simulink model "sysgenIIR_DFormI_dp"  (Simulink 7.6)
settings: Solver=VariableStepDiscrete  SolverMode=SingleTasking  StartTime=0.0  StopTime=20000  RelTol=1e-3
PreLoadFcn:
  | xlrequire('PreLoadFcn')
values from neighbouring files (symbols this model uses):
  Fs = 1 ./ block_data.params.XIncr    [sdspfscope2_r13.m]
undefined symbols (not defined in the file or in its folder): a1, a2, b0, b1, b2, One, sided
libraries: xbsIndex_r4 x46, dspobslib x3, dspsnks4 x3, dspstat3 x2, simulink x2, xbsCopyrightNotice_r4 x1, dspswit3 x1, dspsrcs4 x1
settings Model: Creator=alexc  LastModifiedBy=douangp
settings DataIOCC: SignalLoggingName=sigsOut
settings OptimizationCC: BlockReduction=off  BooleanDataType=off  InlineInvariantSignals=on  InitFltsAndDblsToZero=on
settings DebuggingCC: SaveWithParameterizedLinksMsg=none  SignalResolutionControl=TryResolveAllWithWarning  SolverPrmCheckMsg=none  MultiTaskDSMMsg=warning  MultiTaskCondExecSysMsg=none  StrictBusMsg=None
settings HardwareCC: TargetUnknown=on
settings RTWCC: IncludeERTFirstTime=on
settings GRTTargetCC: TargetFcnLib=ansi_tfl_tmw.mat

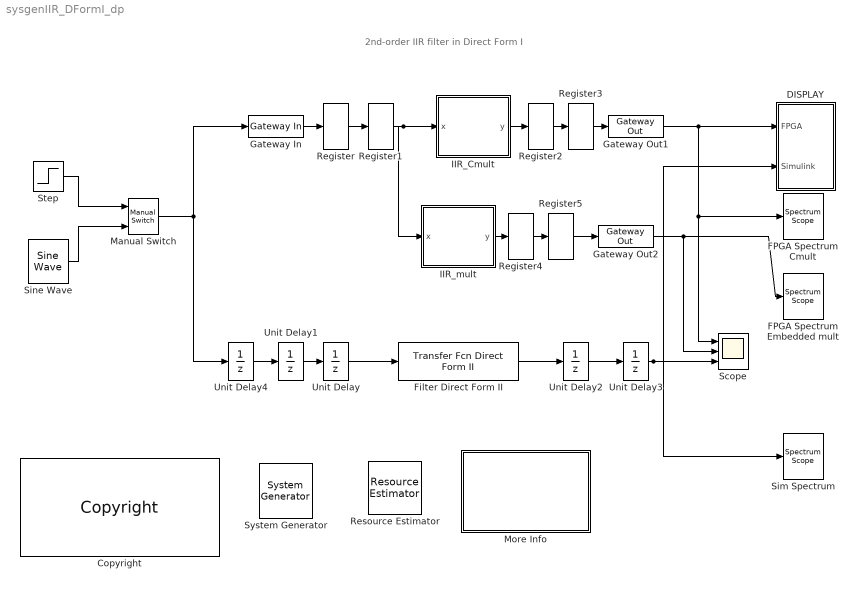
== system sysgenIIR_DFormI_dp ==
  note: 2nd-order IIR filter in Direct Form I
  " System Generator" : xbsIndex_r4/ System Generator  Tag=genX  SystemSampleTime=-1  xilinxfamily=virtex6  part=xc6vlx240t  speed=-1  package=ff1156  synthesis_tool=XST  clock_wrapper=Clock Enables  directory=./sysgenIIR_DFormI_work_registered  testbench=on  simulink_period=Fs  sysclk_period=16  dcm_input_clock_period=100  incr_netlist=off  trim_vbits=According to Block Masks  dbl_ovrd=According to Block Masks  core_generation=According to Block Masks  run_coregen=off  deprecated_control=off  eval_field=0  block_type=sysgen
      settings: block_version=9.2.00
  Copyright : xbsCopyrightNotice_r4/Copyright  copyrighttext="Copyright (c) 2010  by  Xilinx, Inc. All rights reserved.<br><br>This file contains proprietary, confidential information of Xilinx, Inc., is distributed under license from Xilinx, Inc., and may be used, copied and/or disclosed only pursuant to the terms of a valid license agreement with Xilinx, Inc. Xilinx hereby grants you a license to use this file solely for design, simulation, implementation and creation of design files limited to Xilinx devices or technologies. Use with non-Xilinx devices or technologies is expressly prohibited and immediately terminates your license unless covered by a separate agreement.<br><br>Xilinx is providing this design, code, or information \"as-is\" solely for use in developing programs and solutions for Xilinx devices, with no obligation on the part of Xilinx to provide support. By providing this design, code, or information as one possible implementation of this feature, application or standard, Xilinx is making no representation that this implementation is free from any claims of infringement. You are responsible for obtaining any rights you may require for your implementation. Xilinx expressly disclaims any warranty whatsoever with respect to the adequacy of the implementation, including but not limited to any warranties or representations that this implementation is free from claims of infringement, implied warranties of merchantability or fitness for a particular purpose.<br><br>Xilinx products are not intended for use in life support appliances, devices, or systems. Use in such applications is expressly prohibited.<br><br>Any modifications that are made to the Source Code are done at the user's sole risk and will be unsupported.<br><br>This copyright and support notice must be retained as part of this text at all times. (c) Copyright 1995-2010 Xilinx, Inc. All rights reserved."  block_type=copyright
      settings: block_version=10.1.00
      settings: infoedit=|
      | Copyright(C) 2008 by  Xilinx, Inc. All rights reserved.<br>
      | <br>
      | This file contains proprietary, confidential information of Xilinx, Inc., is distributed under license
      | from Xilinx, Inc., and may be used, copied and/or disclosed only pursuant to the terms of a valid license
      | agreement with Xilinx, Inc. Xilinx hereby grants you a license to use this file solely for design,
      | simulation, implementation and creation of design files limited to Xilinx devices or technologies. Use
      | with non-Xilinx devices or technologies is expressly prohibited and immediately terminates your license
      | unless covered by a separate agreement.<br>
      | <br>
      | Xilinx is providing this design, code, or information "as-is" solely for use in developing programs and
      | solutions for Xilinx devices, with no obligation on the part of Xilinx to provide support. By providing
      | this design, code, or information as one possible implementation of this feature, application or standard,
      | Xilinx is making no representation that this implementation is free from any claims of infringement. You
      | are responsible for obtaining any rights you may require for your implementation. Xilinx expressly disclaims
      | any warranty whatsoever with respect to the adequacy of the implementation, including but not limited to any
      | warranties or representations that this implementation is free from claims of infringement, implied warranties
      | of merchantability or fitness for a particular purpose.<br>
      | <br>
      | Xilinx products are not intended for use in life support appliances, devices, or systems. Use in such
      | applications is expressly prohibited.<br>
      | <br>
      | Any modifications that are made to the Source Code are done at the user's sole risk and will be unsupported.<br>
      | <br>
      | This copyright and support notice must be retained as part of this text at all times.
      | (c) Copyright 1995-2008 Xilinx, Inc. All rights reserved.
  DISPLAY : Subsystem  TreatAsAtomicUnit=on
  FPGA Spectrum Cmult : dspsnks4/Spectrum Scope  DialogController=dspdialog.SpectrumScope  DialogControllerArgs=DataTag5  SystemSampleTime=-1  ScopeProperties=off  Domain=Frequency  HorizSpan=1  UseBuffer=on  BufferSize=512  Overlap=0  inpFftLenInherit=off  FFTlength=128  numAvg=10  DisplayProperties=off  AxisGrid=on  Memory=off  FrameNumber=on  AxisLegend=off  AxisZoom=off  OpenScopeAtSimStart=on  OpenScopeImmediately=off  FigPos=[465 290 423 236]  AxisProperties=off  XUnits=Hertz  XRange=One-sided ([0...Fs/2])  XDisplay=0  InheritXIncr=on  XIncr=1.0  XLabel=Samples  XLimit=Auto  YUnits=dBW/Hertz  XMax=1  XMin=0  YLabel=Magnitude, dB  LineProperties=off  LineColors=[0.1 0.2 0.7]|[0.6 0.2 0.1]|[0.1 0.6 0.1]  wintypeSpecScope=Hann  RsSpecScope=50  betaSpecScope=5  winsampSpecScope=Periodic  XAxisParamsVer=6.8
      settings: YMin=-150  YMax=20
  FPGA Spectrum Embedded mult : dspsnks4/Spectrum Scope  DialogController=dspdialog.SpectrumScope  DialogControllerArgs=DataTag6  SystemSampleTime=-1  ScopeProperties=off  Domain=Frequency  HorizSpan=1  UseBuffer=on  BufferSize=512  Overlap=0  inpFftLenInherit=off  FFTlength=128  numAvg=1  DisplayProperties=off  AxisGrid=on  Memory=off  FrameNumber=on  AxisLegend=off  AxisZoom=off  OpenScopeAtSimStart=on  OpenScopeImmediately=off  FigPos=[1105 390 423 236]  AxisProperties=off  XUnits=Hertz  XRange=One-sided ([0...Fs/2])  XDisplay=0  InheritXIncr=on  XIncr=1.0  XLabel=Samples  XLimit=Auto  YUnits=dBW/Hertz  XMax=1  XMin=0  YLabel=Magnitude, dB  LineProperties=off  LineColors=[0.1 0.2 0.7]|[0.6 0.2 0.1]|[0.1 0.6 0.1]  wintypeSpecScope=Hann  RsSpecScope=50  betaSpecScope=5  winsampSpecScope=Periodic  XAxisParamsVer=6.9
      settings: YMin=-150  YMax=20
  Filter Direct Form II : simulink/Additional Math & Discrete/Additional Discrete/Transfer Fcn Direct Form II  SystemSampleTime=-1  NumCoefVec=[1 -1.6929 1]  DenCoefVec=[1.2591 0.82538]  vinit=0.0  DoSatur=off
  Gateway In : xbsIndex_r4/Gateway In  arith_type="Signed  (2's comp)"  n_bits=data_width  bin_pt=data_binary_pt  quantization="Round  (unbiased: +/- Inf)"  overflow=Saturate  period=Fs  dbl_ovrd=off  timing_constraint=None  locs_specified=off  LOCs={}  hdl_port=on  block_type=gatewayin
      settings: infoedit="Gateway in block.  Converts inputs of type Simulink integer, double and fixed point to  Xilinx fixed point type.<P><P>Hardware notes:  In hardware these blocks become top level input ports."  xl_area=[0 0 0 0 12 0 0]  block_version=VER_STRING_GOES_HERE
  Gateway Out1 : xbsIndex_r4/Gateway Out  hdl_port=on  timing_constraint=None  locs_specified=off  LOCs={}  block_type=gatewayout
      settings: infoedit="Gateway out block.  Converts Xilinx fixed point inputs into ouputs of type Simulink integer, double, or fixed point.<P><P>Hardware notes:  In hardware these blocks become top level output ports or are discarded, depending on how they are configured."  xl_area=[0 0 0 0 12 0 0]  block_version=VER_STRING_GOES_HERE
  Gateway Out2 : xbsIndex_r4/Gateway Out  hdl_port=on  timing_constraint=None  locs_specified=off  LOCs={}  block_type=gatewayout
      settings: infoedit="Gateway out block.  Converts Xilinx fixed point inputs into ouputs of type Simulink integer, double, or fixed point.<P><P>Hardware notes:  In hardware these blocks become top level output ports or are discarded, depending on how they are configured."  xl_area=[0 0 0 0 12 0 0]  block_version=VER_STRING_GOES_HERE
  IIR_Cmult : Subsystem
  IIR_mult : Subsystem
  Manual Switch : simulink/Signal Routing/Manual Switch  SystemSampleTime=-1  sw=0  action=0  varsize=off
  More Info : Subsystem
      mask Display: disp('Double click\n for\n more information.')
  Register{,1..5} (6 alike) : xbsIndex_r4/Register  init=0  rst=off  en=off  dbl_ovrd=off  block_type=register
      settings: block_version=VER_STRING_GOES_HERE
  Resource Estimator : xbsIndex_r4/Resource Estimator  Tag=resEstTag  Slices=307  FFs=120  BRAMs=0  LUTs=476  IOBs=36  EBMs=5  TBUFs=0  xl_use_estimator_area=off  est_options=Estimate  xl_estimator_area=[307 120 0 476 36 5 0]  mrp_directory=./sysgenIIR_DFormI_work  simulink_period=Fs  block_type=resource_estimator
      settings: AttributesFormatString=Resource\nEstimator  block_version=9.2.00
  Scope : Scope  NumInputPorts=3
      settings: YMin=-5~-5~-5  YMax=5~5~5
  Sim Spectrum : dspsnks4/Spectrum Scope  DialogController=dspdialog.SpectrumScope  DialogControllerArgs=DataTag7  SystemSampleTime=-1  ScopeProperties=off  Domain=Frequency  HorizSpan=1  UseBuffer=on  BufferSize=512  Overlap=0  inpFftLenInherit=off  FFTlength=128  numAvg=10  DisplayProperties=on  AxisGrid=on  Memory=off  FrameNumber=on  AxisLegend=off  AxisZoom=off  OpenScopeAtSimStart=on  OpenScopeImmediately=off  FigPos=[465 290 423 236]  AxisProperties=off  XUnits=Hertz  XRange=One-sided ([0...Fs/2])  XDisplay=0  InheritXIncr=on  XIncr=1.0  XLabel=Samples  XLimit=Auto  YUnits=dBW/Hertz  XMax=1  XMin=0  YLabel=Magnitude, dB  LineProperties=off  LineColors=[0.1 0.2 0.7]|[0.6 0.2 0.1]|[0.1 0.6 0.1]  wintypeSpecScope=Hann  RsSpecScope=50  betaSpecScope=5  winsampSpecScope=Periodic  XAxisParamsVer=6.8
      settings: YMin=-150  YMax=20
  Sine Wave : dspsrcs4/Sine Wave  Amplitude=0.99  Frequency=1/32  Phase=0  SampleMode=Discrete  OutComplex=Real  CompMethod=Trigonometric fcn  TableSize=Speed  SampleTime=1/Fs  SamplesPerFrame=1  ResetState=Restart at time zero  dataType=double  wordLen=16  udDataType=sfix(16)  fracBitsMode=Best precision  numFracBits=14  OutDataTypeStr=double  LastOutDataTypeStr=double
  Step : Step  Before=1  After=0  SampleTime=1
  Unit Delay{,1..4} (5 alike) : UnitDelay  SampleTime=Fs
  wires:
  Gateway In/1 -> Register/1
  Gateway Out1/1 -> FPGA Spectrum Cmult/1, Scope/1, DISPLAY/1(FPGA)
  Unit Delay/1 -> Filter Direct Form II/1
  IIR_Cmult/1(y) -> Register2/1
  Filter Direct Form II/1 -> Unit Delay2/1
  Gateway Out2/1 -> Scope/2, FPGA Spectrum Embedded mult/1
  Sine Wave/1 -> Manual Switch/2
  Step/1 -> Manual Switch/1
  Manual Switch/1 -> Gateway In/1, Unit Delay4/1
  Register/1 -> Register1/1
  Register1/1 -> IIR_Cmult/1(x), IIR_mult/1(x)
  Register2/1 -> Register3/1
  Register3/1 -> Gateway Out1/1
  Register4/1 -> Register5/1
  IIR_mult/1(y) -> Register4/1
  Register5/1 -> Gateway Out2/1
  Unit Delay1/1 -> Unit Delay/1
  Unit Delay2/1 -> Unit Delay3/1
  Unit Delay3/1 -> Scope/3, DISPLAY/2(Simulink), Sim Spectrum/1
  Unit Delay4/1 -> Unit Delay1/1

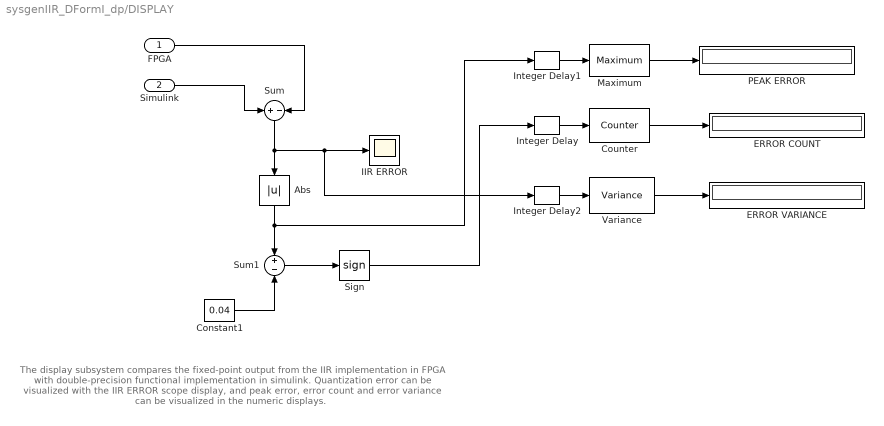
== system sysgenIIR_DFormI_dp/DISPLAY ==
  note: The display subsystem compares the fixed-point output from the IIR implementation in FPGA
      | with double-precision functional implementation in simulink. Quantization error can be visualized
      | with the IIR ERROR scope display, and peak error, error count and error variance can be visualized
      | in the numeric displays.
  FPGA : Inport
  Simulink : Inport  Port=2
  Abs : Abs  SaturateOnIntegerOverflow=on
  Constant1 : Constant  Value=0.04
  Counter : dspswit3/Counter  Direction=Up  CountEvent=Rising edge  CounterSize=User defined  MaxCount=200000000  InitialCount=0  Output=Count  HitValue=32  ResetInput=off  SamplesPerFrame=1  Ts=1  CntDtype=double  HitDtype=Logical
  ERROR COUNT : Display
      settings: Format=long_e
  ERROR VARIANCE : Display
      settings: Format=long_e
  IIR ERROR : Scope
      settings: TimeRange=10000  YMin=-0.0006  YMax=0.0005  SaveName=ScopeData2
  Integer Delay : dspobslib/Integer Delay  delay=1  ic=0  reset_popup=None
  Integer Delay1 : dspobslib/Integer Delay  delay=1  ic=0  reset_popup=None
  Integer Delay2 : dspobslib/Integer Delay  delay=1  ic=0  reset_popup=None
  Maximum : dspstat3/Maximum  DialogController=dspDDGCreate  DialogControllerArgs=DataTag2  fcn=Running  reset=None  InputProcessing=Inherited (this choice will be removed - see release notes)  indexBase=One  operateOver=Each column  Dimension=1  colComp=on  operation=maximum  roiEnable=off  roiType=Rectangles  roiPortion=Entire ROI  roiOutput=Individual statistics for each ROI  roiFlag=off  accumDataTypeStr=Inherit: Same as product output  accumLastDataTypeStr=Inherit: Same as product output  roundingMode=Floor  overflowMode=off
  PEAK ERROR : Display
      settings: Format=long_e
  Sign : Signum
  Sum : Sum  Inputs=+-  SaturateOnIntegerOverflow=on  InputSameDT=on  OutDataTypeStr=Inherit: Same as first input
  Sum1 : Sum  Inputs=+-  SaturateOnIntegerOverflow=on  InputSameDT=on  OutDataTypeStr=Inherit: Same as first input
  Variance : dspstat3/Variance  DialogController=dspDDGCreate  DialogControllerArgs=DataTag4  run=on  reset_popup=None  InputProcessing=Inherited (this choice will be removed - see release notes)  directionMode=Each column  dimension=1  treatSBRowAsCol=on  roiEnable=off  roiType=Rectangles  roiPortion=Entire ROI  roiOutput=Individual statistics for each ROI  roiFlag=off  roundingMode=Floor  overflowMode=off
  wires:
  FPGA/1 -> Sum/2
  Simulink/1 -> Sum/1
  Sum/1 -> Abs/1, IIR ERROR/1, Integer Delay2/1
  Constant1/1 -> Sum1/2
  Abs/1 -> Sum1/1, Integer Delay1/1
  Sum1/1 -> Sign/1
  Sign/1 -> Integer Delay/1
  Counter/1 -> ERROR COUNT/1
  Variance/1 -> ERROR VARIANCE/1
  Maximum/1 -> PEAK ERROR/1
  Integer Delay/1 -> Counter/1
  Integer Delay1/1 -> Maximum/1
  Integer Delay2/1 -> Variance/1

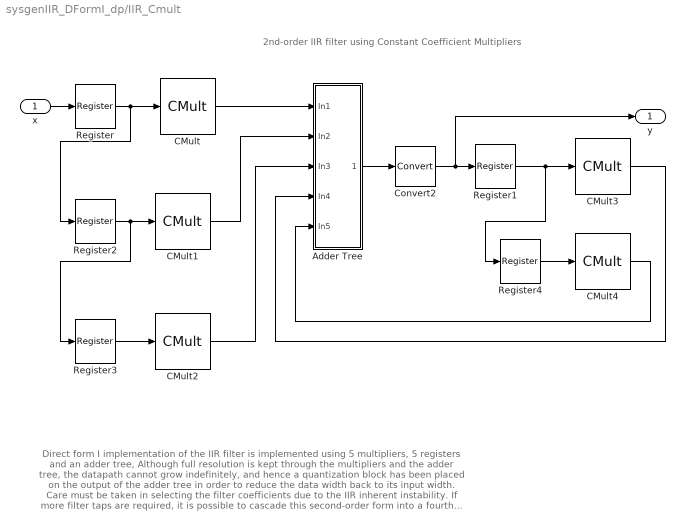
== system sysgenIIR_DFormI_dp/IIR_Cmult ==
  note: Direct form I implementation of the IIR filter is implemented using 5 multipliers, 5 registers
      | and an adder tree, Although full resolution is kept through the multipliers and the
      | adder tree, the datapath cannot grow indefinitely, and hence a quantization block has
      | been placed on the output of the adder tree in order to reduce the data width back to its
      | input width.
      | Care must be taken in selecting the filter coefficients due to the IIR inherent instability.
      |
      | If more filter taps are required, it is possible to cascade this second-order form into a
      | fourth order cascaded filter or combine them in parallel. The advantage of designing
      | filters in this way is that they are modular, which makes their implementation much simpler.
      |
      | In IIR_Cmult, we chose to use constant coefficient multipliers which are very efficiently
      | implemented in LUTs. Partial products are currently saved in distributed memories,
      | but an option in the CMult block allows the user to target Block Memories if necessary.
      | Uses 191 slices and runs at  60 MHz in a XC2V80-6. Because of the feedback loop, no
      | latency and hence no pipelining is possible in this design. It is for this reason, fairly
      | difficult to achieve high sample rate with such implementation. On the other hand, it is
      | possible to reduce the size and performance by processing the data sequentially instead of
      | in parallel as currently shown in this example.
  note: 2nd-order IIR filter using Constant Coefficient Multipliers
  x : Inport
  Adder Tree : Subsystem
  CMult : xbsIndex_r4/CMult  const=b0  const_n_bits=coef_width  const_bin_pt=coef_binary_pt  en=off  latency=0  precision=Full  arith_type="Signed  (2's comp)"  n_bits=8  bin_pt=6  quantization="Round  (unbiased: +/- Inf)"  overflow=Wrap  dbl_ovrd=off  use_behavioral_HDL=off  mem_type=Distributed RAM  pipeline=off  use_rpm=off  placement_style=Rectangular Shape  block_type=cmult
      settings: xl_area=[0 0 0 0 0 0 0]  block_version=VER_STRING_GOES_HERE
  CMult1 : xbsIndex_r4/CMult  const=b1  const_n_bits=coef_width  const_bin_pt=coef_binary_pt  en=off  latency=0  precision=Full  arith_type="Signed  (2's comp)"  n_bits=8  bin_pt=6  quantization="Round  (unbiased: +/- Inf)"  overflow=Wrap  dbl_ovrd=off  use_behavioral_HDL=off  mem_type=Distributed RAM  pipeline=off  use_rpm=off  placement_style=Rectangular Shape  block_type=cmult
      settings: xl_area=[41 0 0 78 0 0 0]  block_version=VER_STRING_GOES_HERE
  CMult2 : xbsIndex_r4/CMult  const=b2  const_n_bits=coef_width  const_bin_pt=coef_binary_pt  en=off  latency=0  precision=Full  arith_type="Signed  (2's comp)"  n_bits=8  bin_pt=6  quantization="Round  (unbiased: +/- Inf)"  overflow=Wrap  dbl_ovrd=off  use_behavioral_HDL=off  mem_type=Distributed RAM  pipeline=off  use_rpm=off  placement_style=Rectangular Shape  block_type=cmult
      settings: xl_area=[0 0 0 0 0 0 0]  block_version=VER_STRING_GOES_HERE
  CMult3 : xbsIndex_r4/CMult  const=-a1  const_n_bits=coef_width  const_bin_pt=coef_binary_pt  en=off  latency=0  precision=Full  arith_type="Signed  (2's comp)"  n_bits=8  bin_pt=6  quantization="Round  (unbiased: +/- Inf)"  overflow=Wrap  dbl_ovrd=off  use_behavioral_HDL=off  mem_type=Distributed RAM  pipeline=off  use_rpm=off  placement_style=Rectangular Shape  block_type=cmult
      settings: xl_area=[42 0 0 83 0 0 0]  block_version=VER_STRING_GOES_HERE
  CMult4 : xbsIndex_r4/CMult  const=-a2  const_n_bits=coef_width  const_bin_pt=coef_binary_pt  en=off  latency=0  precision=Full  arith_type="Signed  (2's comp)"  n_bits=8  bin_pt=6  quantization="Round  (unbiased: +/- Inf)"  overflow=Wrap  dbl_ovrd=off  use_behavioral_HDL=off  mem_type=Distributed RAM  pipeline=off  use_rpm=off  placement_style=Rectangular Shape  block_type=cmult
      settings: xl_area=[42 0 0 83 0 0 0]  block_version=VER_STRING_GOES_HERE
  Convert2 : xbsIndex_r4/Convert  arith_type="Signed  (2's comp)"  n_bits=data_width  bin_pt=data_binary_pt  quantization=Truncate  overflow=Saturate  en=off  latency=0  dbl_ovrd=off  pipeline=off  block_type=convert
      settings: infoedit=The input is presented at the output after quantization and overflow effects.<P><P>Hardware notes: Additional hardware is used when rounding or saturation is selected and output width is less than the input width.  xl_area=[8 0 0 16 0 0 0]  block_version=VER_STRING_GOES_HERE
  Register{,1..4} (5 alike) : xbsIndex_r4/Register  init=0  rst=off  en=off  dbl_ovrd=off  block_type=register
      settings: xl_area=[6 12 0 0 0 0 0]  block_version=VER_STRING_GOES_HERE
  y : Outport
  wires:
  Register/1 -> Register2/1, CMult/1
  Register2/1 -> Register3/1, CMult1/1
  Register3/1 -> CMult2/1
  CMult/1 -> Adder Tree/1(In1)
  CMult1/1 -> Adder Tree/2(In2)
  CMult2/1 -> Adder Tree/3(In3)
  Register4/1 -> CMult4/1
  CMult3/1 -> Adder Tree/4(In4)
  CMult4/1 -> Adder Tree/5(In5)
  Adder Tree/1(Out1) -> Convert2/1
  Register1/1 -> Register4/1, CMult3/1
  x/1 -> Register/1
  Convert2/1 -> Register1/1, y/1

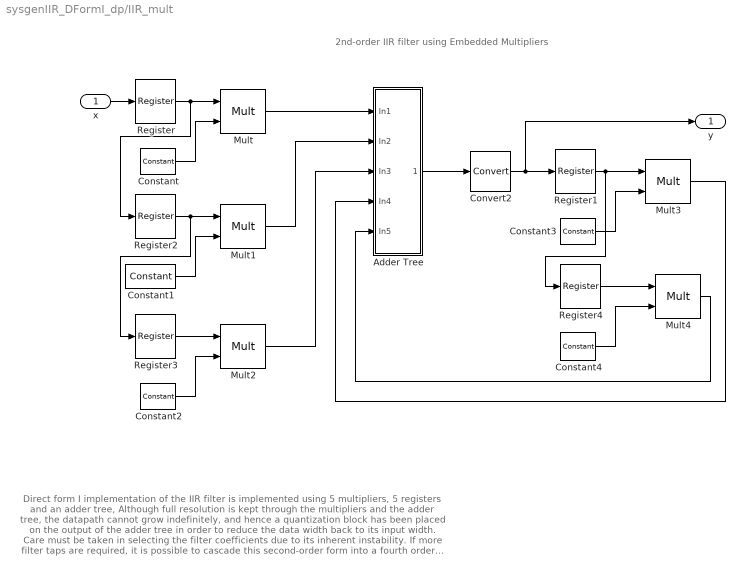
== system sysgenIIR_DFormI_dp/IIR_mult ==
  note: Direct form I implementation of the IIR filter is implemented using 5 multipliers, 5 registers
      | and an adder tree, Although full resolution is kept through the multipliers and the
      | adder tree, the datapath cannot grow indefinitely, and hence a quantization block has
      | been placed on the output of the adder tree in order to reduce the data width back to its
      | input width.
      | Care must be taken in selecting the filter coefficients due to its inherent instability.
      |
      | If more filter taps are required, it is possible to cascade this second-order form into a
      | fourth order cascaded filter, combine them in parallel or time share the current design
      | by saving multiple sets of coefficients in distributed memories. Similarly, the time sharing
      | approach can be used for multi-channel requirements, in which case, the coefficients can
      | be saved in distributed memories or block memories depending on the number of channels.
      |
      | In IIR_mult, we chose to use Virtex-II/Virtex-II Pro embedded multipliers.
      | Uses 87 slices, 5 embedded multipliers and run at 62 MHz in a XC2V80-6.
      | Because of the feedback loop, no latency and hence no pipelining is possible in this design.
      | It is for this reason, fairly difficult to achieve high sample rate with such implementation.
  note: 2nd-order IIR filter using Embedded Multipliers
  x : Inport
  Adder Tree : Subsystem
  Constant : xbsIndex_r4/Constant  arith_type=Signed (2's comp)  const=b0  n_bits=coef_width  bin_pt=coef_binary_pt  explicit_period=off  period=1  equ=P=C  opselect=C  inp2=PCIN>>17  opr=+  inp1=P  carry=CIN  dbl_ovrd=off  block_type=constant
      settings: block_version=VER_STRING_GOES_HERE
  Constant1 : xbsIndex_r4/Constant  arith_type=Signed (2's comp)  const=b1  n_bits=coef_width  bin_pt=coef_binary_pt  explicit_period=off  period=1  equ=P=C  opselect=C  inp2=PCIN>>17  opr=+  inp1=P  carry=CIN  dbl_ovrd=off  block_type=constant
      settings: block_version=VER_STRING_GOES_HERE
  Constant2 : xbsIndex_r4/Constant  arith_type=Signed (2's comp)  const=b2  n_bits=coef_width  bin_pt=coef_binary_pt  explicit_period=off  period=1  equ=P=C  opselect=C  inp2=PCIN>>17  opr=+  inp1=P  carry=CIN  dbl_ovrd=off  block_type=constant
      settings: block_version=VER_STRING_GOES_HERE
  Constant3 : xbsIndex_r4/Constant  arith_type=Signed (2's comp)  const=-a1  n_bits=coef_width  bin_pt=coef_binary_pt  explicit_period=off  period=1  equ=P=C  opselect=C  inp2=PCIN>>17  opr=+  inp1=P  carry=CIN  dbl_ovrd=off  block_type=constant
      settings: block_version=VER_STRING_GOES_HERE
  Constant4 : xbsIndex_r4/Constant  arith_type=Signed (2's comp)  const=-a2  n_bits=coef_width  bin_pt=coef_binary_pt  explicit_period=off  period=1  equ=P=C  opselect=C  inp2=PCIN>>17  opr=+  inp1=P  carry=CIN  dbl_ovrd=off  block_type=constant
      settings: block_version=VER_STRING_GOES_HERE
  Convert2 : xbsIndex_r4/Convert  arith_type="Signed  (2's comp)"  n_bits=data_width  bin_pt=data_binary_pt  quantization=Truncate  overflow=Saturate  en=off  latency=0  dbl_ovrd=off  pipeline=off  block_type=convert
      settings: infoedit=The input is presented at the output after quantization and overflow effects.<P><P>Hardware notes: Additional hardware is used when rounding or saturation is selected and output width is less than the input width.  xl_area=[8 0 0 16 0 0 0]  block_version=VER_STRING_GOES_HERE
  Mult{,1..4} (5 alike) : xbsIndex_r4/Mult  precision=Full  arith_type="Signed  (2's comp)"  n_bits=8  bin_pt=2  quantization=Truncate  overflow=Wrap  en=off  latency=0  dbl_ovrd=off  use_behavioral_HDL=off  opt=Speed  use_embedded=on  optimum_pipeline=off  pipeline=off  use_rpm=off  placement_style=Rectangular shape  block_type=mult
      settings: infoedit=Multiplies two values.<P><P>Hardware notes: To use the internal pipeline stage of the dedicated multiplier you must select 'Pipeline to Greatest Extent Possible'.  xl_area=[0 0 0 0 0 1 0]  block_version=VER_STRING_GOES_HERE
  Register{,1..4} (5 alike) : xbsIndex_r4/Register  init=0  rst=off  en=off  dbl_ovrd=off  block_type=register
      settings: xl_area=[6 12 0 0 0 0 0]  block_version=VER_STRING_GOES_HERE
  y : Outport
  wires:
  x/1 -> Register/1
  Register1/1 -> Mult3/1, Register4/1
  Constant3/1 -> Mult3/2
  Convert2/1 -> y/1, Register1/1
  Mult4/1 -> Adder Tree/5(In5)
  Mult3/1 -> Adder Tree/4(In4)
  Constant4/1 -> Mult4/2
  Register4/1 -> Mult4/1
  Mult2/1 -> Adder Tree/3(In3)
  Constant2/1 -> Mult2/2
  Register3/1 -> Mult2/1
  Constant1/1 -> Mult1/2
  Register2/1 -> Register3/1, Mult1/1
  Constant/1 -> Mult/2
  Register/1 -> Register2/1, Mult/1
  Mult1/1 -> Adder Tree/2(In2)
  Mult/1 -> Adder Tree/1(In1)
  Adder Tree/1(Out1) -> Convert2/1

== system sysgenIIR_DFormI_dp/More Info ==
  note: This design example shows two distinct FPGA implementations of a 2nd order IIR filter in Direct Form I,
      | and compares them to the double precision Simulink IIR filter block.
      |
      | IIR_Cmult is implemented using constant coefficient multipliers implemented in LUTs
      |
      | IIR_mult is implemented using embedded multipliers. This approach can only be used
      | with the FPGAs that provide the embedded multipliers.
      |
      | Multiple display blocks allow the user to visualize the Power Spectrum  Density (PSD) of each
      | implementation as well as the quantization error in the DISPLAY block.
      |
      | All the variables such as data width, coefficient width, Sample period, and coefficient values are
      | initialized in the sysgenIIR_PreLoadFcn.m file. The default setting use 12 bit data and coefficients
  note: 2nd-order IIR filter in Direct Form I

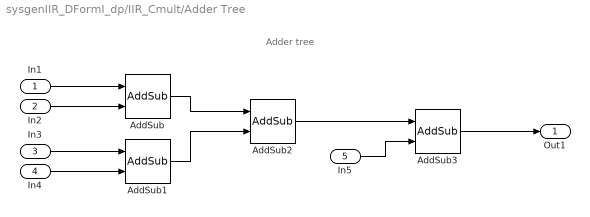
== system sysgenIIR_DFormI_dp/IIR_Cmult/Adder Tree ==
  note: Adder tree
  In1 : Inport
  In2 : Inport  Port=2
  In3 : Inport  Port=3
  In4 : Inport  Port=4
  In5 : Inport  Port=5
  AddSub : xbsIndex_r4/AddSub  mode=Addition  use_carryin=off  use_carryout=off  en=off  latency=0  precision=Full  arith_type=Unsigned  n_bits=8  bin_pt=2  quantization=Truncate  overflow=Wrap  dbl_ovrd=off  use_behavioral_HDL=off  hw_selection=Fabric  pipelined=off  use_rpm=off  block_type=addsub
      settings: xl_area=[13 0 0 25 0 0 0]  block_version=VER_STRING_GOES_HERE
  AddSub1 : xbsIndex_r4/AddSub  mode=Addition  use_carryin=off  use_carryout=off  en=off  latency=0  precision=Full  arith_type=Unsigned  n_bits=8  bin_pt=2  quantization=Truncate  overflow=Wrap  dbl_ovrd=off  use_behavioral_HDL=on  hw_selection=Fabric  pipelined=off  use_rpm=off  block_type=addsub
      settings: xl_area=[13 0 0 24 0 0 0]  block_version=VER_STRING_GOES_HERE
  AddSub2 : xbsIndex_r4/AddSub  mode=Addition  use_carryin=off  use_carryout=off  en=off  latency=0  precision=Full  arith_type=Unsigned  n_bits=8  bin_pt=2  quantization=Truncate  overflow=Wrap  dbl_ovrd=off  use_behavioral_HDL=on  hw_selection=Fabric  pipelined=off  use_rpm=off  block_type=addsub
      settings: xl_area=[13 0 0 25 0 0 0]  block_version=VER_STRING_GOES_HERE
  AddSub3 : xbsIndex_r4/AddSub  mode=Addition  use_carryin=off  use_carryout=off  en=off  latency=0  precision=Full  arith_type=Unsigned  n_bits=8  bin_pt=2  quantization=Truncate  overflow=Wrap  dbl_ovrd=off  use_behavioral_HDL=off  hw_selection=Fabric  pipelined=off  use_rpm=off  block_type=addsub
      settings: xl_area=[14 0 0 26 0 0 0]  block_version=VER_STRING_GOES_HERE
  Out1 : Outport
  wires:
  In1/1 -> AddSub/1
  In2/1 -> AddSub/2
  In5/1 -> AddSub3/2
  AddSub3/1 -> Out1/1
  In3/1 -> AddSub1/1
  In4/1 -> AddSub1/2
  AddSub/1 -> AddSub2/1
  AddSub1/1 -> AddSub2/2
  AddSub2/1 -> AddSub3/1

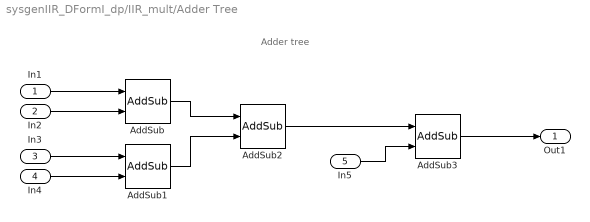
== system sysgenIIR_DFormI_dp/IIR_mult/Adder Tree ==
  note: Adder tree
  In1 : Inport
  In2 : Inport  Port=2
  In3 : Inport  Port=3
  In4 : Inport  Port=4
  In5 : Inport  Port=5
  AddSub : xbsIndex_r4/AddSub  mode=Addition  use_carryin=off  use_carryout=off  en=off  latency=0  precision=Full  arith_type=Unsigned  n_bits=8  bin_pt=2  quantization=Truncate  overflow=Wrap  dbl_ovrd=off  use_behavioral_HDL=off  hw_selection=Fabric  pipelined=off  use_rpm=off  block_type=addsub
      settings: xl_area=[13 0 0 25 0 0 0]  block_version=VER_STRING_GOES_HERE
  AddSub1 : xbsIndex_r4/AddSub  mode=Addition  use_carryin=off  use_carryout=off  en=off  latency=0  precision=Full  arith_type=Unsigned  n_bits=8  bin_pt=2  quantization=Truncate  overflow=Wrap  dbl_ovrd=off  use_behavioral_HDL=on  hw_selection=Fabric  pipelined=off  use_rpm=off  block_type=addsub
      settings: xl_area=[13 0 0 24 0 0 0]  block_version=VER_STRING_GOES_HERE
  AddSub2 : xbsIndex_r4/AddSub  mode=Addition  use_carryin=off  use_carryout=off  en=off  latency=0  precision=Full  arith_type=Unsigned  n_bits=8  bin_pt=2  quantization=Truncate  overflow=Wrap  dbl_ovrd=off  use_behavioral_HDL=on  hw_selection=Fabric  pipelined=off  use_rpm=off  block_type=addsub
      settings: xl_area=[13 0 0 25 0 0 0]  block_version=VER_STRING_GOES_HERE
  AddSub3 : xbsIndex_r4/AddSub  mode=Addition  use_carryin=off  use_carryout=off  en=off  latency=0  precision=Full  arith_type=Unsigned  n_bits=8  bin_pt=2  quantization=Truncate  overflow=Wrap  dbl_ovrd=off  use_behavioral_HDL=off  hw_selection=Fabric  pipelined=off  use_rpm=off  block_type=addsub
      settings: xl_area=[14 0 0 26 0 0 0]  block_version=VER_STRING_GOES_HERE
  Out1 : Outport
  wires:
  In1/1 -> AddSub/1
  In2/1 -> AddSub/2
  In5/1 -> AddSub3/2
  AddSub3/1 -> Out1/1
  In3/1 -> AddSub1/1
  In4/1 -> AddSub1/2
  AddSub/1 -> AddSub2/1
  AddSub1/1 -> AddSub2/2
  AddSub2/1 -> AddSub3/1
